simulink model "hcu_main"  (R2021b)
settings: Solver=FixedStepDiscrete  StartTime=0.0  StopTime=10.0  FixedStep=double(C_TICK_TIME_S)  RelTol=1e-3  EnableMultiTasking=on
values from neighbouring files (symbols this model uses):
  C_TASK_5MS_S = (	C_TICK_TIME_S      	)    [hcu_local_hdr.m]
libraries: hal x2, app x1, inp x1, outp x1
settings Model: Creator=jc19  LastModifiedBy=B0292
settings SolverCC: AlgebraicLoopSolver=TrustRegion
settings DataIOCC: LimitDataPoints=on  SaveFormat=Array  SignalLoggingSaveFormat=ModelDataLogs  ReturnWorkspaceOutputs=off
settings OptimizationCC: DefaultParameterBehavior=Inlined  ExpressionDepthLimit=2147483647  InitFltsAndDblsToZero=on  LifeSpan=inf
settings DebuggingCC: CheckSSInitialOutputMsg=off  UnderspecifiedInitializationDetection=Classic  MergeDetectMultiDrivingBlocksExec=none  SolverPrmCheckMsg=warning  ParameterPrecisionLossMsg=none  FcnCallInpInsideContextMsg=warning  SignalLabelMismatchMsg=warning  StateNameClashWarn=warning  SFUnexpectedBacktrackingDiag=warning  SFNoUnconditionalDefaultTransitionDiag=warning  SFExecutionAtInitializationDiag=none  SFMachineParentedDataDiag=warning  ArithmeticOperatorsInVariantConditions=warning
settings HardwareCC: ProdBitPerPointer=32  ProdBitPerSizeT=32  ProdBitPerPtrDiffT=32  ProdLargestAtomicFloat=None  ProdIntDivRoundTo=Undefined  ProdEndianess=Unspecified  ProdWordSize=32  ProdHWDeviceType=32-bit Generic
settings ModelReferenceCC: PropagateSignalLabelsOutOfModel=off
settings SFSimCC: SimUseLocalCustomCode=off  CustomCodeUndefinedFunction=UseInterfaceOnly
settings RTWCC: RTWUseLocalCustomCode=off
settings CodeAppCC: StateflowObjectComments=on
settings GRTTargetCC: TargetLangStandard=C89/C90 (ANSI)  CombineOutputUpdateFcns=off  GRTInterface=on
settings ConfigComp: CovMetricSettings=dw  CovSaveCumulativeToWorkspaceVar=on  CovSaveSingleToWorkspaceVar=on  CovExternalEMLEnable=off

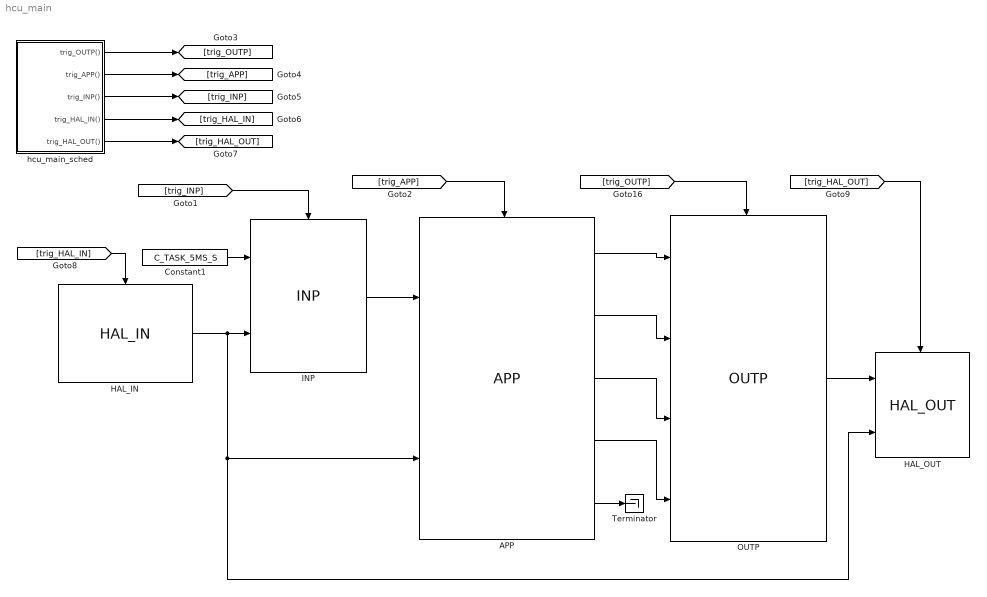
== system hcu_main ==
  APP : app/APP  SystemSampleTime=-1  VariantActivationTime=update diagram  Latency=0  AutoFrameSizeCalculation=off
  Constant1 : Constant  Value=C_TASK_5MS_S  OutDataTypeStr=single
  HAL_IN : hal/HAL_IN  SystemSampleTime=-1  VariantActivationTime=update diagram  Latency=0  AutoFrameSizeCalculation=off
  HAL_OUT : hal/HAL_OUT  SystemSampleTime=-1  VariantActivationTime=update diagram  Latency=0  AutoFrameSizeCalculation=off
  INP : inp/INP  SystemSampleTime=-1  VariantActivationTime=update diagram  Latency=0  AutoFrameSizeCalculation=off
  OUTP : outp/OUTP  SystemSampleTime=-1  VariantActivationTime=update diagram  Latency=0  AutoFrameSizeCalculation=off
  Terminator : Terminator
  hcu_main_sched : Stateflow chart  TreatAsAtomicUnit=on
  wires:
  hcu_main_sched/1(trig_OUTP()) -> [trig_OUTP]
  hcu_main_sched/2(trig_APP()) -> [trig_APP]
  hcu_main_sched/3(trig_INP()) -> [trig_INP]
  [trig_INP] -> INP/Trigger
  [trig_OUTP] -> OUTP/Trigger
  [trig_APP] -> APP/Trigger
  INP/1 -> APP/1
  OUTP/1 -> HAL_OUT/1
  HAL_IN/1 -> INP/2, HAL_OUT/2, APP/2
  Constant1/1 -> INP/1
  hcu_main_sched/4(trig_HAL_IN()) -> [trig_HAL_IN]
  hcu_main_sched/5(trig_HAL_OUT()) -> [trig_HAL_OUT]
  [trig_HAL_IN] -> HAL_IN/Trigger
  [trig_HAL_OUT] -> HAL_OUT/Trigger
  APP/1 -> OUTP/1
  APP/2 -> OUTP/2
  APP/3 -> OUTP/3
  APP/4 -> OUTP/4
  APP/5 -> Terminator/1

== stateflow chart hcu_main/hcu_main_sched ==
  (default) -> (junction 2) : {
      |     trig_HAL_IN;
      |     trig_INP;
      |     trig_APP;
      |     trig_OUTP;
      |     trig_HAL_OUT;
      | }
  events: trig_OUTP output FUNCTION_CALL_EVENT; trig_APP output FUNCTION_CALL_EVENT; trig_INP output FUNCTION_CALL_EVENT; trig_HAL_IN output FUNCTION_CALL_EVENT; trig_HAL_OUT output FUNCTION_CALL_EVENT
